simulink model "ConfiguredVirtualVehicleModel"  (R2025b)
settings: Solver=daessc  StartTime=0  StopTime=2474  FixedStep=.001  RelTol=1e-2  EnableMultiTasking=on
StopFcn:
  | %toc
undefined symbols (not defined in the file or in its folder): AccelOvrCmd, CtrlTcuInitGear, DecelOvrCmd, Disabled, DriverPreviewDist, EnblAccelOvr, EnblDecelCmd, EnblSteerCmd, EnvAbsPrs, EnvAirTemp, EnvGrvty, EnvNomFrictionScaling, EnvNominalGrade, EnvWindVelX, EnvWindVelY, EnvWindVelZ, FTP75, MotoFrmInert, MotoFrmLngth, MotoFrmMass, MotoLowrFrntFrkMass, MotoRearArmLngth, MotoRearArmMass, MotoUpprFrntFrkMass, RiderLkAhdPtDstGain, RiderMass, ScnAccTbl, ScnBrkTbl, ScnCRMaxLatAccel, ScnCRRadius, ScnDLCGateLongPos, ScnDLCLatRef, ScnDLCLatRefOffset, ScnDLCLongRefBpt, ScnDLCLongRefStartPos, ScnDLCVehicleWidth, ScnFHCounterDwellTime, ScnFHInitialDwellTime, ScnFHReturnTime, ScnFHRollRateZeroCross, ScnFHSteerAmp, ScnFHSteerSpeed, ScnISHandwheelRate, ScnISMaxHandwheelAng, ScnISMaxLatAccel, ScnISSteerHoldTime, ScnLongPosBpts, ScnLongVelRef, ScnOvalTrackl, ScnOvalTrackpdst, ScnOvalTrackr, ScnSDDwellTime, ScnSDSteerAmp, ScnSDSteerFreq, ScnSSFinalFreq, ScnSSSteerAmp, ScnSSSweepTime, ScnStartTime, ScnStrgAngTbl, ScnStrgTrqTbl ... (+10)
libraries: simulink x16, vehdynlibscenariocommon x9, sm_lib x6, autolibshared x4, nesl_utility x4, vehdynlibviscommon x3, sim3dgroundtruthsensorlib x2, vehdynlibdriver x2, sharedtransform x1, autolibutils x1, sim3dautolib x1, sim3dlib x1
(part 4 of 6)

== system ConfiguredVirtualVehicleModel/Rider Commands/Rider Commands/Roll angle control ==
  MotoFdbk : Inport
  MotoRef : Inport  Port=2
  GearCmd : Inport  Port=3
  Bus Creator1 : BusCreator  Inputs=5
  Bus Selector : BusSelector  OutputSignals=MSteer
  Bus Selector1 : BusSelector  OutputSignals=SteerOvrCmd,AccelOvrCmd,DecelOvrCmd
  Constant : Constant  Value=false
  Constant1 : Constant  Value=30*pi/180
  Demux : Demux  Outputs=1
  Equal Front Rear Bias : Selector  InputPortWidth=1  IndexOptions=Index vector (dialog)  Indices=[1 1]  OutputSizes=1
  Gain : Gain
  Mux : Mux  Inputs=1
  Rider Steering Control : Subsystem  mask{RiderControlTypePanel=Roll angle control, TrajectoryTypePanel=Oval, RidTrajContG=0.11, RidTrajContGphi=-21.5, RidTrajContGphid=9, RidTrajContGl=1.7, RidTrajContTD=0.1, RidTrajContTL=0.1, RidRollContGphi=-21.5, RidRollContGphid=9, Trajr=15, Trajl=80, Trajpointdist=1, TrajDatFile='Traj.mat'}
      mask prompts: RiderControlTypePanel "Rider control type:"; TrajectoryTypePanel "Trajectory type:"; RidTrajContG "Gain to determine the Target roll angle, RidContG [rad/m]:"; RidTrajContGphi "Gain to follow the Target trajectory, RidContGphi [Nm/rad]:"; RidTrajContGphid "Gain to prevent the vehicle from tipping over, RidContGphid [Nms/rad]:"; RidTrajContGl "Gain that determines the distance to the look ahead point, RidContGl [s]:"; RidTrajContTD "Time constant for 1st order delay, RidContTD [s]:"; RidTrajContTL "Dead time of rider operation, RidContTL [s]:"; RidRollContGphi "Gain to follow the Target trajectory, RidContGphi [Nm/rad]:"; RidRollContGphid "Gain to prevent the vehicle from tipping over, RidContGphid [Nms/rad]:"; Trajr "Trajectory parameter,Trajr [m]:"; Trajl "Trajectory parameter,Trajl [m]:"; Trajpointdist "Trajpdist [m]:"; TrajDatFile "Trajectory data file:"
      mask init:
      | maskObj = Simulink.Mask.get(gcb);
      | 
      | Type_tmp = maskObj.getParameter('RiderControlTypePanel');
      | Type     = Type_tmp.Value;
      | 
      | TrajGroup = maskObj.getDialogControl('RiderTrajectoryControlParamPanel');
      | RollGroup = maskObj.getDialogControl('RiderRollControlParamPanel');
      | 
      | TrajectoryTypePanel = maskObj.getDialogControl('TrajectoryTypeCont');
      | TargetTrajectoryParamGroup = maskObj.getDialogControl('TargetTrajectoryParamGroup');
      | 
      | GroupAll = maskObj.getDialogControl('RiderControlParamGroup');
      | 
      | switch Type
      |     case 'Roll angle control'
      |     TrajGroup.Visible = 'off';
      |     RollGroup.Visible = 'on';
      |     GroupAll.Visible = 'on';
      |     TrajectoryTypePanel.Visible = 'off';
      |     TargetTrajectoryParamGroup.Visible = 'off';
      |     InputConnector('TargetRollAngle','on');
      |     case 'Target trajectory driving - Look ahead point'
      |     TrajGroup.Visible = 'on';
      |     RollGroup.Visible = 'off';
      |     GroupAll.Visible = 'on';
      |     TrajectoryTypePanel.Visible = 'on';
      |     TargetTrajectoryParamGroup.Visible = 'on';
      |     InputConnector('TargetRollAngle','off','Ground');
      | end
      | 
      | switch Type
      |     case 'Oval'
      | % ------------------------------------------------------------------------%
      | %  Create Trajectory
      | % ------------------------------------------------------------------------%
      | % --- Oval --- %
      | % top part %
      | x_straight1 = -Trajl/2:Trajpointdist:Trajl/2;
      | y_straight1 = x_straight1*0;
      | 
      | % bottom part %
      | x_straight2 = -Trajl/2:Trajpointdist:Trajl/2;
      | y_straight2 = x_straight1*0+2*Trajr;
      | 
      | % right part %
      | theta_corner1 = -pi/2:Trajpointdist/Trajr:pi/2;
      | x_corner1     = Trajr*cos(theta_corner1)+Trajl/2;
      | y_corner1     = Trajr*sin(theta_corner1)+Trajr;
      | 
      | % left part %
      | theta_corner2 = pi/2:Trajpointdist/Trajr:3/2*pi;
      | x_corner2     = Trajr*cos(theta_corner2)-Trajl/2;
      | y_corner2     = Trajr*sin(theta_corner2)+Trajr;
      | 
      | % total %
      | x_oval = [x_straight1, x_corner1(2:end), fliplr(x_straight2), x_corner2(2:end)];
      | y_oval = [y_straight1, y_corner1(2:end), fliplr(y_straight2), y_corner2(2:end)];
      | 
      | trackData(1,:) = x_oval;
      | trackData(2,:) = y_oval;
      | trackData(3,:) = y_oval*0;
      | 
      |     case 'User defined'
      | 
      | TmpTraj = load(TrajDatFile);
      | 
      | trackData(1,:) = TmpTraj.TrajX;
      | trackData(2,:) = -TmpTraj.TrajY;
      | trackData(3,:) = TmpTraj.TrajY*0;
      | 
      | end
      mask Callback RiderControlTypePanel:
      | maskObj = Simulink.Mask.get(gcb);
      | 
      | Type_tmp = maskObj.getParameter('RiderControlTypePanel');
      | Type     = Type_tmp.Value;
      | 
      | TrajGroup = maskObj.getDialogControl('RiderTrajectoryControlParamPanel');
      | RollGroup = maskObj.getDialogControl('RiderRollControlParamPanel');
      | 
      | TrajectoryTypePanel = maskObj.getDialogControl('TrajectoryTypeCont');
      | TargetTrajectoryParamGroup = maskObj.getDialogControl('TargetTrajectoryParamGroup');
      | 
      | GroupAll = maskObj.getDialogControl('RiderControlParamGroup');
      | 
      | switch Type
      |     case 'Roll angle control'
      |     set_param([gcb,'/Rider Steering'],'RiderControlTypePanel','Roll angle control')
      |     TrajGroup.Visible = 'off';
      |     RollGroup.Visible = 'on';
      |     GroupAll.Visible = 'on';
      |     TrajectoryTypePanel.Visible = 'off';
      |     TargetTrajectoryParamGroup.Visible = 'off';
      |     InputConnector('TargetRollAngle','on');
      |     case 'Target trajectory driving - Look ahead point'
      |     set_param([gcb,'/Rider Steering'],'RiderControlTypePanel','Target trajectory driving - Look ahead point')
      |     TrajGroup.Visible = 'on';
      |     RollGroup.Visible = 'off';
      |     GroupAll.Visible = 'on';
      |     TrajectoryTypePanel.Visible = 'on';
      |     TargetTrajectoryParamGroup.Visible = 'on';
      |     InputConnector('TargetRollAngle','off','Ground');
      | end
      mask TypeOptions TrajectoryTypePanel: Oval | User defined
      mask Callback TrajectoryTypePanel:
      | maskObj = Simulink.Mask.get(gcb);
      | 
      | Type_tmp = maskObj.getParameter('TrajectoryTypePanel');
      | Type = Type_tmp.Value;
      | 
      | TargetTrajectoryParamOvalPanel = maskObj.getDialogControl('TargetTrajectoryParamOvalPanel');
      | 
      | TargetTrajectoryParamUserDefinedPanel = maskObj.getDialogControl('TargetTrajectoryParamUserDefinedPanel');
      | 
      | TargetTrajectoryParamGroup = maskObj.getDialogControl('TargetTrajectoryParamGroup');
      | 
      | switch Type
      |     case 'Oval'
      |         set_param([gcb,'/Rider Steering'],'TrajectoryTypePanel','Oval')
      |         % TargetTrajectoryParamGroup.Visible = 'on';
      |         TargetTrajectoryParamOvalPanel.Visible = 'on';
      |         TargetTrajectoryParamUserDefinedPanel.Visible = 'off';
      |     case 'User defined'
      |     set_param([gcb,'/Rider Steering'],'TrajectoryTypePanel','User defined')
      |         % TargetTrajectoryParamGroup.Visible = 'on';
      |         TargetTrajectoryParamOvalPanel.Visible = 'off';
      |         TargetTrajectoryParamUserDefinedPanel.Visible = 'on';
      | end
      mask DialogControl RiderOptionsGroup Prompt: Options
      mask DialogControl RiderTrajectoryControlParamPanel Prompt: Control parameters
      mask DialogControl RiderRollControlParamPanel Prompt: Control parameters
      mask DialogControl TargetTrajectoryParamOvalPanel Prompt: Trajectory parameters
      mask DialogControl OvalTrajConfBtn Prompt: Confirm
      mask DialogControl OvalTrajConfBtn Callback:
      | maskObj = Simulink.Mask.get(gcb);
      | 
      | Trajr_tmp          = maskObj.getParameter('Trajr');
      | Trajr              = str2num(Trajr_tmp.Value);
      | Trajl_tmp          = maskObj.getParameter('Trajl');
      | Trajl              = str2num(Trajl_tmp.Value);
      | Trajpointdist_tmp  = maskObj.getParameter('Trajpointdist');
      | Trajpointdist      = str2num(Trajpointdist_tmp.Value);
      | 
      | % ------------------------------------------------------------------------%
      | %  Create Trajectory
      | % ------------------------------------------------------------------------%
      | % --- Oval --- %
      | % top part %
      | x_straight1 = -Trajl/2:Trajpointdist:Trajl/2;
      | y_straight1 = x_straight1*0;
      | 
      | % bottom part %
      | x_straight2 = -Trajl/2:Trajpointdist:Trajl/2;
      | y_straight2 = x_straight1*0+2*Trajr;
      | 
      | % right part %
      | theta_corner1 = -pi/2:Trajpointdist/Trajr:pi/2;
      | x_corner1     = Trajr*cos(theta_corner1)+Trajl/2;
      | y_corner1     = Trajr*sin(theta_corner1)+Trajr;
      | 
      | % left part %
      | theta_corner2 = pi/2:Trajpointdist/Trajr:3/2*pi;
      | x_corner2     = Trajr*cos(theta_corner2)-Trajl/2;
      | y_corner2     = Trajr*sin(theta_corner2)+Trajr;
      | 
      | % total %
      | x_oval = [x_straight1, x_corner1(2:end), fliplr(x_straight2), x_corner2(2:end)];
      | y_oval = [y_straight1, y_corner1(2:end), fliplr(y_straight2), y_corner2(2:end)];
      | 
      | figure;
      | plot(x_oval, -y_oval);
      | axis equal;
      | grid on;
      | xlabel('Coordinate X [m]');
      | ylabel('Coordinate Y [m]');
      | title('Oval target trajectory');
      | set(gca,'YDir','reverse')
      mask DialogControl TargetTrajectoryParamUserDefinedPanel Prompt: Trajectory parameters
      mask DialogControl UserDefinedTrajConfBtn Prompt: Confirm
      mask DialogControl UserDefinedTrajConfBtn Callback:
      | maskObj = Simulink.Mask.get(gcb);
      | 
      | File_tmp = maskObj.getParameter('TrajDatFile');
      | File     = replace(File_tmp.Value,'''','');
      | 
      | TmpTraj = load(File);
      | 
      | figure;
      | plot(TmpTraj.TrajX, TmpTraj.TrajY);
      | grid on;
      | axis equal;
      | xlabel('Coordinate X [m]');
      | ylabel('Coordinate Y [m]');
      | title('User defined target trajectory');
      | set(gca,'YDir','reverse');
  Signal Specification{,1..3} (4 alike) : SignalSpecification  Unit=1
  Signal Specification4 : SignalSpecification  Unit=N*m
  Terminator : Terminator
  Rider : Outport  VectorParamsAs1DForOutWhenUnconnected=off
  wires:
  Signal Specification2/1 -> Bus Creator1/4  "GearCmd"
  Bus Selector1/3 -> Signal Specification1/1  "<DecelOvrCmd>"
  Bus Creator1/1 -> Rider/1
  Bus Selector1/2 -> Signal Specification/1  "<AccelOvrCmd>"
  MotoFdbk/1 -> Rider Steering Control/1(sensors)
  Signal Specification/1 -> Bus Creator1/2  "AccelCmd"
  Equal Front Rear Bias/1 -> Bus Creator1/3  "DecelCmd"
  Constant/1 -> Bus Creator1/5  "IgnSwtch"
  MotoRef/1 -> Bus Selector1/1
  GearCmd/1 -> Signal Specification2/1
  Bus Selector1/1 -> Signal Specification3/1  "<SteerOvrCmd>"
  Rider Steering Control/1(RiderInfo) -> Bus Selector/1  "SteerCmd"
  Signal Specification1/1 -> Equal Front Rear Bias/1  "DecelCmd"
  Bus Selector/1 -> Mux/1  "<MSteer>"
  Mux/1 -> Demux/1
  Signal Specification4/1 -> Bus Creator1/1  "SteerCmd"
  Signal Specification3/1 -> Terminator/1  "SteerCmd"
  Constant1/1 -> Rider Steering Control/2(TargetRollAngle)
  Gain/1 -> Signal Specification4/1
  Demux/1 -> Gain/1  "SteerCmd"

== system ConfiguredVirtualVehicleModel/Rider Commands/Rider Commands/Target trajectory following - Look ahead point ==
  MotoFdbk : Inport
  MotoRef : Inport  Port=2
  Env : Inport  Port=3
  Bus Creator1 : BusCreator  Inputs=5
  Bus Selector : BusSelector  OutputSignals=MSteer
  Bus Selector1 : BusSelector  OutputSignals=SteerOvrCmd,LngRef,EnblAccelOvr,AccelOvrCmd,AccelHld,AccelZero,EnblDecelCmd,DecelOvrCmd,DecelHld,DecelZero
  Bus Selector2 : BusSelector  OutputSignals=Body.BdyFrm.Cg.Vel.xdot
  Bus Selector3 : BusSelector  OutputSignals=Grade
  Constant : Constant  Value=false
  Demux : Demux  Outputs=1
  Equal Front Rear Bias : Selector  InputPortWidth=1  IndexOptions=Index vector (dialog)  Indices=[1 1]  OutputSizes=1
  Gain : Gain
  Longitudinal Driver : autolibshared/Longitudinal Driver  extAccelOvr=on  extDecelOvr=on  extAccelHld=on  extDecelHld=on  extAccelZero=on  extDecelZero=on  cntrlType=Predictive  shftType=Reverse, Neutral, Drive  velUnits=m/s  gearOut=on  Kp=5  Ki=5  Kff=.1  Kg=0  VehVelVec=[0 100]  KffVec=[.1 .1]  KpVec=[10 10]  KiVec=[5 5]  KgVec=[0 0]  m=MotoFrmMass+MotoUpprFrntFrkMass+MotoLowrFrntFrkMass+MotoRearArmMass+RiderMass  Kpt=DriverTractiveForce  tau=DriverTimeConst  L=DriverPreviewDist  aR=DriverRollRes  bR=DriverDrivelineRes  cR=DriverAeroRes  g=EnvGrvty  vnom=5  Kaw=1  tauerr=.1  tauPt=2  GearInit=DriverInitialGear  tShift=DriverShiftTime  pdlVec=[0.1 0.4 0.5 0.9]  upShftTbl=[-1 12.9375 26.4375 39.9375 51.18749999999999 62.4375 72.84375 83.25;-1 16.3125 29.8125 43.3125 54.5624 65.8125 76.78125 87.75;-1 19.6875 33.1875 46.68749999999999 57.9375 69.1875 80.71875 92.25;-1 33 52.5 77.25 100.5 138.75 161.875 185]  dwnShftTbl=[1 9.5625 23.0625 36.5625 47.8125 59.0625 68.90625 78.75;1 12.9375 26.4375 39.9375 51.18749999999999 62.4375 72.84375 83.25;1 16.3125 29.8125 43.3125 54.562499 65.8125 76.78125 87.75;1 19.6875 33.1875 46.68749999999999 57.9375 69.1875 80.71875 92.25]  tClutch=.5  tRev=.5  tPark=120  aMode=6  UpGearVec="[0  1  2  3  4  5  6  7]"  DownGearVec="[1  2  3  4  5  6  7  8]"
  Mux : Mux  Inputs=1
  Rider Steering Control : vehdynlibscenariocommon/Rider Steering Control  RiderControlTypePanel=Target trajectory driving - Look ahead point  RidTrajContG=RiderTrgtRollAngGain  RidTrajContGphi=RiderTrgtTrajGain  RidTrajContGphid=RiderPrevTipOvrGain  RidTrajContGl=1.7  RidTrajContTD=RiderFrstOdrTimeCnst  RidTrajContTL=RiderOpDeadTime  RidRollContGphi=-21.5  RidRollContGphid=9
  Signal Specification3 : SignalSpecification  Unit=rad
  Signal Specification4 : SignalSpecification  Unit=N*m
  Terminator : Terminator
  Terminator2 : Terminator
  Unit Conversion1 : UnitConversion
  Rider : Outport  VectorParamsAs1DForOutWhenUnconnected=off
  wires:
  Bus Creator1/1 -> Rider/1
  MotoFdbk/1 -> Bus Selector2/1, Rider Steering Control/1
  Longitudinal Driver/2 -> Bus Creator1/2  "AccelCmd"
  Equal Front Rear Bias/1 -> Bus Creator1/3  "DecelCmd"
  Constant/1 -> Bus Creator1/5  "IgnSwtch"
  Bus Selector1/1 -> Signal Specification3/1  "<SteerOvrCmd>"
  Rider Steering Control/1 -> Bus Selector/1  "SteerCmd"
  Longitudinal Driver/3 -> Equal Front Rear Bias/1  "DecelCmd"
  Bus Selector/1 -> Mux/1  "<MSteer>"
  Mux/1 -> Demux/1
  Signal Specification4/1 -> Bus Creator1/1  "SteerCmd"
  Signal Specification3/1 -> Terminator/1  "SteerCmd"
  Bus Selector1/8 -> Longitudinal Driver/7  "<DecelOvrCmd>"
  Bus Selector1/6 -> Longitudinal Driver/5  "<AccelZero>"
  Bus Selector1/4 -> Longitudinal Driver/3  "<AccelOvrCmd>"
  Bus Selector1/10 -> Longitudinal Driver/9  "<DecelZero>"
  Bus Selector1/5 -> Longitudinal Driver/4  "<AccelHld>"
  MotoRef/1 -> Bus Selector1/1, Rider Steering Control/2
  Bus Selector1/2 -> Unit Conversion1/1  "<LngRef>"
  Bus Selector1/7 -> Longitudinal Driver/6  "<EnblDecelCmd>"
  Bus Selector1/3 -> Longitudinal Driver/2  "<EnblAccelOvr>"
  Bus Selector1/9 -> Longitudinal Driver/8  "<DecelHld>"
  Unit Conversion1/1 -> Longitudinal Driver/1
  Longitudinal Driver/4 -> Bus Creator1/4  "GearCmd"
  Longitudinal Driver/1 -> Terminator2/1
  Bus Selector3/1 -> Longitudinal Driver/11  "<Grade>"
  Env/1 -> Bus Selector3/1
  Bus Selector2/1 -> Longitudinal Driver/10  "<xdot>"
  Gain/1 -> Signal Specification4/1
  Demux/1 -> Gain/1

== system ConfiguredVirtualVehicleModel/Rider Commands/Torque Control/AngleToTorque ==
  MotoFdbk : Inport
  RiderInput : Inport  Port=2
  Bus Creator : BusCreator  Inputs=5
  Bus Selector : BusSelector  OutputSignals=Steer.Genrl.Ang.thetasteer
  Bus Selector1 : BusSelector  OutputSignals=SteerCmd
  Bus Selector2 : BusSelector  OutputSignals=AccelCmd,DecelCmd,GearCmd,IgnSwtch
  Torque Control : vehdynlibsteering/Steering System/Steer by Angle  SystemSampleTime=-1  VariantActivationTime=update diagram  EmptyChoice=off  PassThrough=off  PassThroughVariantControl=(default)  EmptyChoiceVariantControl=(default)  AllowFlexibleInterface=on  Latency=0  AutoFrameSizeCalculation=off
  Rider : Outport
  wires:
  Bus Selector/1 -> Torque Control/2  "<thetasteer>"
  MotoFdbk/1 -> Bus Selector/1
  Bus Selector1/1 -> Torque Control/1  "<SteerCmd>"
  RiderInput/1 -> Bus Selector2/1, Bus Selector1/1
  Bus Selector2/1 -> Bus Creator/2  "<AccelCmd>"
  Bus Selector2/2 -> Bus Creator/3  "<DecelCmd>"
  Bus Selector2/3 -> Bus Creator/4  "<GearCmd>"
  Bus Selector2/4 -> Bus Creator/5  "<IgnSwtch>"
  Torque Control/1 -> Bus Creator/1  "SteerCmd"
  Bus Creator/1 -> Rider/1

== system ConfiguredVirtualVehicleModel/Rider Commands/Torque Control/Look ahead point model ==
  MotoFdbk : Inport
  RiderInput : Inport  Port=2
  MotoRef : Inport  Port=3
  Terminator : Terminator
  Terminator1 : Terminator
  Rider : Outport
  wires:
  MotoFdbk/1 -> Terminator/1
  RiderInput/1 -> Rider/1
  MotoRef/1 -> Terminator1/1

== system ConfiguredVirtualVehicleModel/Rider Commands/Torque Control/NoTorqueControl ==
  MotoFdbk : Inport
  RiderInput : Inport  Port=2
  MotoRef : Inport  Port=3
  Terminator : Terminator
  Terminator1 : Terminator
  Rider : Outport
  wires:
  MotoFdbk/1 -> Terminator/1
  RiderInput/1 -> Rider/1
  MotoRef/1 -> Terminator1/1

== system ConfiguredVirtualVehicleModel/Rider Commands/Torque Control/PID Control ==
  MotoFdbk : Inport
  RiderInput : Inport  Port=2
  MotoRef : Inport  Port=3
  Terminator : Terminator
  Terminator1 : Terminator
  Rider : Outport
  wires:
  MotoFdbk/1 -> Terminator/1
  RiderInput/1 -> Rider/1
  MotoRef/1 -> Terminator1/1

== system ConfiguredVirtualVehicleModel/Visualization/ISO 15037-1:2006/Disabled ==
  VehFdbk : Inport
  Terminator1 : Terminator
  wires:
  VehFdbk/1 -> Terminator1/1

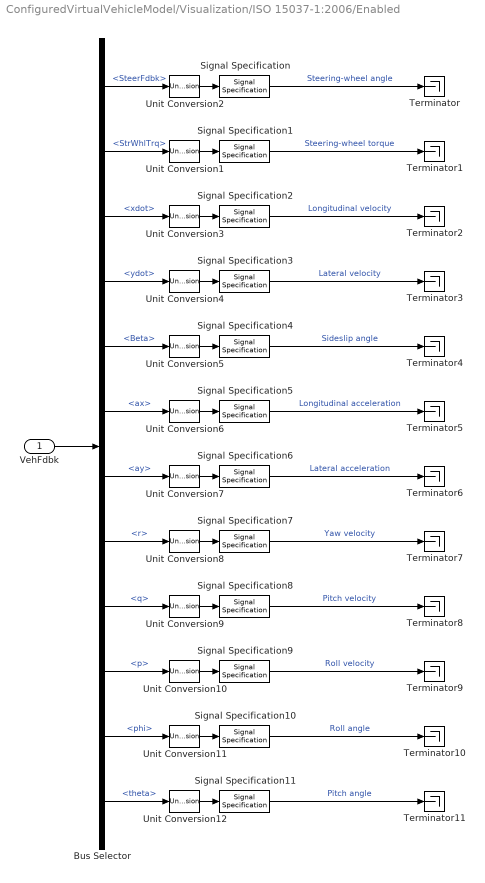
== system ConfiguredVirtualVehicleModel/Visualization/ISO 15037-1:2006/Enabled ==
  VehFdbk : Inport
  Bus Selector : BusSelector  OutputSignals=Rider.SteerFdbk,Steering.StrWhlTrq,Body.BdyFrm.Cg.Vel.xdot,Body.BdyFrm.Cg.Vel.ydot,Body.BdyFrm.Cg.Ang.Beta,Body.BdyFrm.Cg.Acc.ax,Body.BdyFrm.Cg.Acc.ay,Body.BdyFrm.Cg.AngVel.r,Body.BdyFrm.Cg.AngVel.q,Body.BdyFrm.Cg.AngVel.p,Body.InertFrm.Cg.Ang.phi,Body.InertFrm.Cg.Ang.theta
  Signal Specification{,4,10..11} (4 alike) : SignalSpecification  Unit=deg
  Signal Specification1 : SignalSpecification  Unit=N*m
  Signal Specification2 : SignalSpecification  Unit=km/h
  Signal Specification3 : SignalSpecification  Unit=m/s
  Signal Specification5 : SignalSpecification  Unit=m/s^2
  Signal Specification6 : SignalSpecification  Unit=m/s^2
  Signal Specification7 : SignalSpecification  Unit=deg/s
  Signal Specification8 : SignalSpecification  Unit=deg/s
  Signal Specification9 : SignalSpecification  Unit=deg/s
  Terminator{,1..11} (12 alike) : Terminator
  Unit Conversion{1..12} (12 alike) : UnitConversion
  wires:
  Bus Selector/12 -> Unit Conversion12/1  "<theta>"
  Signal Specification11/1 -> Terminator11/1  "Pitch angle"
  Unit Conversion12/1 -> Signal Specification11/1
  Bus Selector/11 -> Unit Conversion11/1  "<phi>"
  Unit Conversion11/1 -> Signal Specification10/1
  Signal Specification10/1 -> Terminator10/1  "Roll angle"
  Bus Selector/10 -> Unit Conversion10/1  "<p>"
  Signal Specification9/1 -> Terminator9/1  "Roll velocity"
  Unit Conversion10/1 -> Signal Specification9/1
  Bus Selector/9 -> Unit Conversion9/1  "<q>"
  Unit Conversion9/1 -> Signal Specification8/1
  Signal Specification8/1 -> Terminator8/1  "Pitch velocity"
  Bus Selector/8 -> Unit Conversion8/1  "<r>"
  Signal Specification7/1 -> Terminator7/1  "Yaw velocity"
  Unit Conversion8/1 -> Signal Specification7/1
  Bus Selector/7 -> Unit Conversion7/1  "<ay>"
  Unit Conversion7/1 -> Signal Specification6/1
  Signal Specification6/1 -> Terminator6/1  "Lateral acceleration"
  Bus Selector/6 -> Unit Conversion6/1  "<ax>"
  Signal Specification5/1 -> Terminator5/1  "Longitudinal acceleration"
  Unit Conversion6/1 -> Signal Specification5/1
  Bus Selector/5 -> Unit Conversion5/1  "<Beta>"
  Unit Conversion5/1 -> Signal Specification4/1
  Signal Specification4/1 -> Terminator4/1  "Sideslip angle"
  Bus Selector/4 -> Unit Conversion4/1  "<ydot>"
  Signal Specification3/1 -> Terminator3/1  "Lateral velocity"
  Unit Conversion4/1 -> Signal Specification3/1
  Bus Selector/3 -> Unit Conversion3/1  "<xdot>"
  Unit Conversion3/1 -> Signal Specification2/1
  Signal Specification2/1 -> Terminator2/1  "Longitudinal velocity"
  Signal Specification1/1 -> Terminator1/1  "Steering-wheel torque"
  Unit Conversion1/1 -> Signal Specification1/1
  Bus Selector/2 -> Unit Conversion1/1  "<StrWhlTrq>"
  Signal Specification/1 -> Terminator/1  "Steering-wheel angle"
  Unit Conversion2/1 -> Signal Specification/1
  VehFdbk/1 -> Bus Selector/1
  Bus Selector/1 -> Unit Conversion2/1  "<SteerFdbk>"

== system ConfiguredVirtualVehicleModel/Visualization/Performance Signal Routing/Performance Calculations ==
  VehSpd : Inport
  FuelVolFlow : Inport  Port=2
  BattPwr : Inport  Port=3
  Add : Sum
  Divide : Product  Inputs=*/
  Divide1 : Product  Inputs=*/
  Divide2 : Product  Inputs=*/
  Integrator : Integrator
  Integrator1 : Integrator
  L/100 Km Calc : Product  Inputs=/*
  Product : Product
  Rate Transition3 : RateTransition  Deterministic=off
  Saturation : Saturate  UpperLimit=Inf  LowerLimit=0.001  ZeroCross=off
  Saturation1 : Saturate  UpperLimit=Inf  LowerLimit=1e-3  ZeroCross=off
  Signal Specification5 : SignalSpecification  Unit=m/s
  Sqrt : Sqrt
  US EPA kwh/USgal equivalent : Constant  Value=33.7
  US MPG Calc : Product  Inputs=*/
  Unit Conversion5 : UnitConversion
  m to 100Km : Gain  Gain=1/1000/100
  m to mile : Gain  Gain=0.000621371
  m^3 per gal : Gain  Gain=0.00378541
  m^3 to L : Gain  Gain=1000
  m^3 to US Gal : Gain  Gain=264.172
  s per h : Constant  Value=3600
  w per kw : Constant  Value=1000
  US MPG : Outport  VectorParamsAs1DForOutWhenUnconnected=off
  L/100Km : Outport  Port=2  VectorParamsAs1DForOutWhenUnconnected=off
  wires:
  m^3 to US Gal/1 -> Saturation1/1
  m^3 to L/1 -> L/100 Km Calc/2
  Integrator/1 -> m to mile/1, m to 100Km/1
  m to mile/1 -> US MPG Calc/1
  FuelVolFlow/1 -> Add/1
  Integrator1/1 -> m^3 to US Gal/1, m^3 to L/1
  Saturation/1 -> L/100 Km Calc/1
  m to 100Km/1 -> Saturation/1
  L/100 Km Calc/1 -> L/100Km/1  "L/100Km"
  US MPG Calc/1 -> Rate Transition3/1
  Saturation1/1 -> US MPG Calc/2
  Rate Transition3/1 -> US MPG/1  "US MPG"
  w per kw/1 -> Divide/2
  Divide/1 -> Divide2/1
  Divide2/1 -> Divide1/1
  s per h/1 -> Divide1/2
  Divide1/1 -> m^3 per gal/1
  Add/1 -> Integrator1/1
  m^3 per gal/1 -> Add/2
  US EPA kwh/USgal equivalent/1 -> Divide2/2
  BattPwr/1 -> Divide/1
  Sqrt/1 -> Integrator/1
  Product/1 -> Sqrt/1
  Signal Specification5/1 -> Product/2, Product/1
  Unit Conversion5/1 -> Signal Specification5/1
  VehSpd/1 -> Unit Conversion5/1

== system ConfiguredVirtualVehicleModel/Visualization/Scope Type/DLC ==
  VehFdbk : Inport
  Vis : Inport  Port=2
  Bus Creator : BusCreator  Inputs=3
  Bus Selector3 : BusSelector  OutputSignals=Body.InertFrm.Cg.Disp.X,Body.InertFrm.Cg.Disp.Z
  Bus Selector4 : BusSelector  OutputSignals=LeftBnd,RightBnd,LtrlRef
  Lane Change : Scope
      settings: Title=Double Lane Change: Lateral Displacement  ActiveDisplayYMinimum=-3.28469  ActiveDisplayYMaximum=6.06905  YLabel=Lateral Displacement [m] (positive = right direction)  DataLoggingSaveFormat=Array
  Mux1 : Mux  Inputs=3
  Rate Transition : RateTransition  OutPortSampleTime=.1
  Rate Transition3 : RateTransition  OutPortSampleTime=.1
  Signal Copy : SignalConversion  OverrideOpt=off
  Signal Copy1 : SignalConversion  OverrideOpt=off
  Signal Copy2 : SignalConversion  OverrideOpt=off
  Ref : Outport  VectorParamsAs1DForOutWhenUnconnected=off
  wires:
  VehFdbk/1 -> Bus Selector3/1
  Vis/1 -> Bus Selector4/1
  Bus Creator/1 -> Ref/1
  Bus Selector3/2 -> Signal Copy2/1  "<Z>"
  Signal Copy/1 -> Bus Creator/2  "YRef"
  Signal Copy1/1 -> Bus Creator/1  "XRef"
  Signal Copy2/1 -> Bus Creator/3  "ZRef"
  Rate Transition3/1 -> Mux1/2  "Right Boundary"
  Bus Selector4/3 -> Signal Copy/1, Mux1/3  "<LtrlRef>"
  Mux1/1 -> Lane Change/1
  Bus Selector4/1 -> Rate Transition/1  "<LeftBnd>"
  Rate Transition/1 -> Mux1/1  "Left Boundary"
  Bus Selector4/2 -> Rate Transition3/1  "<RightBnd>"
  Bus Selector3/1 -> Signal Copy1/1  "<X>"

== system ConfiguredVirtualVehicleModel/Visualization/Scope Type/None ==
  VehFdbk : Inport
  Vis : Inport  Port=2
  Bus Selector2 : BusSelector  OutputSignals=Steer.Genrl.Ang.thetasteer
  Bus Selector9 : BusSelector  OutputSignals=Body.BdyFrm.Cg.AngVel.r
  Signal Specification3 : SignalSpecification  Unit=deg/s
  Unit Conversion4 : UnitConversion
  Yaw Rate and Steer : Scope  NumInputPorts=2
      settings: ActiveDisplayYMinimum=-112.49987  ActiveDisplayYMaximum=112.49996
  Ref : Outport  VectorParamsAs1DForOutWhenUnconnected=off
  wires:
  Bus Selector9/1 -> Unit Conversion4/1  "<r>"
  Signal Specification3/1 -> Yaw Rate and Steer/1
  Unit Conversion4/1 -> Signal Specification3/1
  VehFdbk/1 -> Bus Selector2/1, Bus Selector9/1  "VehFdbk"
  Bus Selector2/1 -> Yaw Rate and Steer/2  "<thetasteer>"
  Vis/1 -> Ref/1

== system ConfiguredVirtualVehicleModel/Visualization/Scope Type/XYZ ==
  VehFdbk : Inport
  Vis : Inport  Port=2
  Terminator : Terminator
  Ref : Outport  VectorParamsAs1DForOutWhenUnconnected=off
  wires:
  Vis/1 -> Ref/1
  VehFdbk/1 -> Terminator/1

== system ConfiguredVirtualVehicleModel/Visualization/Vehicle XY Plotter/Disabled ==

== system ConfiguredVirtualVehicleModel/Visualization/Vehicle XY Plotter/XY View ==
  Bus Element In2 : Inport  PortName=VehFdbk
  Bus Selector1 : BusSelector  OutputSignals=Body.InertFrm.Cg.Ang.phi,Body.InertFrm.Cg.Ang.theta,Body.InertFrm.Cg.Ang.psi  OutputAsBus=on
  Bus Selector2 : BusSelector  OutputSignals=Wheels.FrontTire.Fx,Wheels.RearTire.Fx
  Bus Selector3 : BusSelector  OutputSignals=Wheels.FrontTire.Fy,Wheels.RearTire.Fy
  Bus Selector5 : BusSelector  OutputSignals=Wheels.FrontTire.Alpha,Wheels.RearTire.Alpha
  Bus Selector6 : BusSelector  OutputSignals=Body.InertFrm.Cg.Disp.X,Body.InertFrm.Cg.Disp.Y,Body.InertFrm.Cg.Disp.Z  OutputAsBus=on
  Bus Selector7 : BusSelector  OutputSignals=Body.InertFrm.Cg.Vel.Xdot,Body.InertFrm.Cg.Vel.Ydot,Body.InertFrm.Cg.Vel.Zdot  OutputAsBus=on
  Bus Selector9 : BusSelector  OutputSignals=Driveline.EngSpd,Driveline.EMSpd,Driveline.Gear
  Bus to Vector : BusToVector
  Bus to Vector1 : BusToVector
  Bus to Vector2 : BusToVector
  Max : MinMax  Function=max  Inputs=2
  Multi-Track XY Plotter : vehdynlibviscommon/Multi-Track XY Plotter  numTrack=Single track  extRef=off  extStats=on  extTireF=on  a=1.5  b=1.5  w=0  figBorder=10  bufferSize=1024  velNorm=5  tireFNorm=1000  pltDT=.1
      settings: LibrarySourceBlock=vehdynlibviscommon/Vehicle XY Plot Configuration
  Mux{,1..3} (4 alike) : Mux  Inputs=2
  Unary Minus : UnaryMinus
  wires:
  Bus Selector7/1 -> Bus to Vector1/1
  Bus to Vector1/1 -> Multi-Track XY Plotter/3
  Bus Selector2/1 -> Mux1/1  "<Fx>"
  Bus Selector1/1 -> Bus to Vector2/1
  Bus Selector9/1 -> Max/1  "<EngSpd>"
  Bus to Vector/1 -> Multi-Track XY Plotter/1
  Bus Selector6/1 -> Bus to Vector/1
  Bus to Vector2/1 -> Multi-Track XY Plotter/2
  Bus Element In2/1 -> Bus Selector3/1, Bus Selector2/1, Bus Selector9/1, Bus Selector5/1, Bus Selector7/1, Bus Selector1/1, Bus Selector6/1  "VehFdbk"
  Mux3/1 -> Multi-Track XY Plotter/4
  Mux1/1 -> Multi-Track XY Plotter/6
  Mux2/1 -> Unary Minus/1
  Max/1 -> Mux/1
  Bus Selector9/2 -> Max/2  "<EMSpd>"
  Mux/1 -> Multi-Track XY Plotter/5
  Bus Selector9/3 -> Mux/2  "<Gear>"
  Bus Selector2/2 -> Mux1/2  "<Fx>"
  Bus Selector3/2 -> Mux2/2  "<Fy>"
  Bus Selector3/1 -> Mux2/1  "<Fy>"
  Bus Selector5/1 -> Mux3/1  "<Alpha>"
  Bus Selector5/2 -> Mux3/2  "<Alpha>"
  Unary Minus/1 -> Multi-Track XY Plotter/7

== system ConfiguredVirtualVehicleModel/Visualization/Vehicle XY Plotter/XY View Ref ==
  Bus Element In2 : Inport  PortName=VehFdbk
  Bus Element In1 : Inport  Port=2  PortName=Ref  Element=YRef
  Bus Element In3 : Inport  Port=2  PortName=Ref  Element=XRef
  Bus Selector1 : BusSelector  OutputSignals=Body.InertFrm.Cg.Ang.phi,Body.InertFrm.Cg.Ang.theta,Body.InertFrm.Cg.Ang.psi  OutputAsBus=on
  Bus Selector10 : BusSelector  OutputSignals=Wheels.FrontTire.Fx,Wheels.RearTire.Fx,Wheels.FrontTire.Fy,Wheels.RearTire.Fy
  Bus Selector5 : BusSelector  OutputSignals=Steer.Genrl.Ang.thetasteer,Wheels.RearTire.Alpha
  Bus Selector6 : BusSelector  OutputSignals=Body.InertFrm.Cg.Disp.X,Body.InertFrm.Cg.Disp.Y,Body.InertFrm.Cg.Disp.Z  OutputAsBus=on
  Bus Selector7 : BusSelector  OutputSignals=Body.InertFrm.Cg.Vel.Xdot,Body.InertFrm.Cg.Vel.Ydot,Body.InertFrm.Cg.Vel.Zdot  OutputAsBus=on
  Bus Selector9 : BusSelector  OutputSignals=Driveline.EngSpd,Driveline.EMSpd,Driveline.Gear
  Bus to Vector : BusToVector
  Bus to Vector1 : BusToVector
  Bus to Vector2 : BusToVector
  Ground1 : Ground
  Max : MinMax  Function=max  Inputs=2
  Multi-Track XY Plotter : vehdynlibviscommon/Multi-Track XY Plotter  numTrack=Single track  extRef=on  extStats=on  extTireF=on  a=1.5  b=1.5  w=0  figBorder=10  bufferSize=1024  velNorm=5  tireFNorm=1000  pltDT=.1
      settings: LibrarySourceBlock=vehdynlibviscommon/Vehicle XY Plot Configuration
  Mux : Mux  Inputs=3
  Mux{1..4} (4 alike) : Mux  Inputs=2
  Unary Minus : UnaryMinus
  wires:
  Bus Selector7/1 -> Bus to Vector1/1
  Ground1/1 -> Mux/3
  Mux2/1 -> Unary Minus/1
  Bus to Vector1/1 -> Multi-Track XY Plotter/3
  Mux1/1 -> Multi-Track XY Plotter/7
  Bus Selector1/1 -> Bus to Vector2/1
  Bus Element In1/1 -> Mux/2
  Mux4/1 -> Multi-Track XY Plotter/6
  Bus Element In3/1 -> Mux/1
  Mux/1 -> Multi-Track XY Plotter/5
  Bus to Vector/1 -> Multi-Track XY Plotter/1
  Bus Selector6/1 -> Bus to Vector/1
  Bus to Vector2/1 -> Multi-Track XY Plotter/2
  Bus Selector5/1 -> Mux3/1  "<thetasteer>"
  Mux3/1 -> Multi-Track XY Plotter/4
  Bus Selector5/2 -> Mux3/2  "<Alpha>"
  Bus Selector10/1 -> Mux1/1  "<Fx>"
  Bus Selector10/2 -> Mux1/2  "<Fx>"
  Bus Selector10/3 -> Mux2/1  "<Fy>"
  Bus Selector10/4 -> Mux2/2  "<Fy>"
  Unary Minus/1 -> Multi-Track XY Plotter/8
  Bus Selector9/3 -> Mux4/2  "<Gear>"
  Bus Selector9/1 -> Max/1  "<EngSpd>"
  Bus Selector9/2 -> Max/2  "<EMSpd>"
  Max/1 -> Mux4/1
  Bus Element In2/1 -> Bus Selector9/1, Bus Selector10/1, Bus Selector5/1, Bus Selector7/1, Bus Selector1/1, Bus Selector6/1  "VehFdbk"

== system ConfiguredVirtualVehicleModel/Environment/Friction/Varying Friction/Road Track Friction ==
  XWhl : Inport
  YWhl : Inport  Port=2
  Cg : Inport  Port=3
  2D Lookup Tbl for Scaling Fctr (Lambda) : Subsystem  TreatAsAtomicUnit=on
      mask init:
      | [~]=vehdynicon('vehdynblk',gcb);
  Bus Selector : BusSelector  OutputSignals=X,Y
  Cnst Lambda : Constant  Value=ones(2,1).*lambda_g
  Constant1 : Constant  Value=SplitLambdaTrck
  Creating Inertial Frm Bpt : Subsystem
  En at t = 0 : Subsystem
  "Lambda (t = 0) " : Memory  InitialCondition=ones(2,1).*lambda_g  InheritSampleTime=on
  Switch : Switch  Criteria=u2 > Threshold  ZeroCross=off  SaturateOnIntegerOverflow=off  InputSameDT=off
  FricCoeffLambda : Outport
  wires:
  YWhl/1 -> 2D Lookup Tbl for Scaling Fctr (Lambda)/2(YWhl)
  XWhl/1 -> 2D Lookup Tbl for Scaling Fctr (Lambda)/1(XWhl)
  2D Lookup Tbl for Scaling Fctr (Lambda)/1(Lambda for each whl) -> Switch/1
  "Lambda (t = 0) "/1 -> FricCoeffLambda/1
  Switch/1 -> "Lambda (t = 0) "/1
  Cnst Lambda/1 -> Switch/3
  Constant1/1 -> Switch/2
  Cg/1 -> Bus Selector/1
  Creating Inertial Frm Bpt/1(XBpt) -> 2D Lookup Tbl for Scaling Fctr (Lambda)/3(XBpt)
  Creating Inertial Frm Bpt/2(YBpt) -> 2D Lookup Tbl for Scaling Fctr (Lambda)/4(YBpt)
  Bus Selector/1 -> Creating Inertial Frm Bpt/1(XCg)  "<X>"
  Bus Selector/2 -> Creating Inertial Frm Bpt/2(YCg)  "<Y>"
  En at t = 0/1(Out1) -> Creating Inertial Frm Bpt/Enable

== system ConfiguredVirtualVehicleModel/Environment/Friction/Varying Friction/Wheel Coordinates ==
  FrntAxlX : Inport
  RearAxlX : Inport  Port=2
  FrntAxlY : Inport  Port=3
  RearAxlY : Inport  Port=4
  Matrix Concatenate : Concatenate  Mode=Multidimensional array
  Matrix Concatenate1 : Concatenate  Mode=Multidimensional array
  XWhl : Outport
  YWhl : Outport  Port=2
  wires:
  Matrix Concatenate/1 -> XWhl/1
  FrntAxlX/1 -> Matrix Concatenate/1
  Matrix Concatenate1/1 -> YWhl/1
  FrntAxlY/1 -> Matrix Concatenate1/1
  RearAxlY/1 -> Matrix Concatenate1/2
  RearAxlX/1 -> Matrix Concatenate/2

== system ConfiguredVirtualVehicleModel/Environment/Ground Feedback/3D Engine/3D Engine Source ==
  WheelFdbk : Inport
  Multiple Points : Subsystem  VariantControl=terrType==2
  Single Point : Subsystem  VariantControl=terrType ==1
  z : Outport
  DCM : Outport  Port=2

== system ConfiguredVirtualVehicleModel/Motorcycle Vehicle/Hand Levers and Pedals/Hand Levers and Pedals/Brake Pedal ==
  DecelCmd : Inport
  Dead Zone1 : DeadZone  LowerValue=0  UpperValue=.01  ZeroCross=off
  DecelFdbk : Outport
  wires:
  Dead Zone1/1 -> DecelFdbk/1
  DecelCmd/1 -> Dead Zone1/1

== system ConfiguredVirtualVehicleModel/Motorcycle Vehicle/Transmission, Driveline and Brakes/Transmission and Driveline/Driveline ==
  FCpR : Inport
  ThetaFrm : Inport  Port=2
  ThetaArmR : Inport  Port=3
  MBrkR : Inport  Port=4
  AngAWhlR : Inport  Port=5
  DrvSprktTrq : Inport  Port=6
  Chain_Drive : Subsystem  VariantControl=Chain_Drive  ReferencedSubsystem=Chain_Drive
  Info : Outport
  DrvSprktSpd : Outport  Port=2

== system ConfiguredVirtualVehicleModel/Motorcycle Vehicle/Transmission, Driveline and Brakes/Transmission and Driveline/Transmission ==
  EngTrq : Inport
  GearCmd : Inport  Port=2
  EMTrq : Inport  Port=3
  DrvSprktSpd : Inport  Port=4
  ConventionalMotorcycle : Subsystem  VariantControl=ConventionalMotorcycle  ReferencedSubsystem=ConventionalMotorcycle
  EngSpd : Outport
  Gear : Outport  Port=2
  EMSpd : Outport  Port=3
  DrvSprktTrq : Outport  Port=4

== system ConfiguredVirtualVehicleModel/Reference Generator for Motorcycle/3D Engine/3D Engine/Wheel Rotations ==
  MotoFdbk : Inport
  Bus Selector2 : BusSelector  OutputSignals=Wheels.FrontTire.Omega,Wheels.RearTire.Omega
  Constant{4,6..8} (4 alike) : Constant  Value=0  VectorParams1D=off
  Demux : Demux  Outputs=2
  Integrator : Integrator  WrapState=on  WrappedStateUpperValue=2*pi  WrappedStateLowerValue=0  ZeroCross=off
  Mux1 : Mux  Inputs=2
  Rotation : Concatenate  NumInputs=3  Mode=Multidimensional array  ConcatenateDimension=2
  Rotation1 : Concatenate  NumInputs=3  Mode=Multidimensional array  ConcatenateDimension=2
  Front : Outport
  Rear : Outport  Port=2
  wires:
  Constant4/1 -> Rotation1/1
  Mux1/1 -> Integrator/1
  Integrator/1 -> Demux/1
  Demux/1 -> Rotation/2
  Demux/2 -> Rotation1/2
  Constant7/1 -> Rotation/1
  Constant8/1 -> Rotation/3
  Constant6/1 -> Rotation1/3
  Bus Selector2/1 -> Mux1/1  "<Omega>"
  Rotation1/1 -> Rear/1
  Bus Selector2/2 -> Mux1/2  "<Omega>"
  Rotation/1 -> Front/1
  MotoFdbk/1 -> Bus Selector2/1

== system ConfiguredVirtualVehicleModel/Reference Generator for Motorcycle/Reference Router/Steering Command Override/Control Signals ==
  note: 1) Add Subsystem or Model blocks as valid variant choices.
      | 2) You cannot connect blocks at this level. At simulation, connectivity is automatically
      | determined, based on the active variant and port name matching.
  Time : Inport
  Position : Inport  Port=2
  Position-Based Angle : Subsystem  VariantControl=OverrideType==2 && ActType== 2
  Position-Based Torque : Subsystem  VariantControl=OverrideType==1 && ActType== 2
  Time-Based Angle : Subsystem  VariantControl=OverrideType==2 && ActType==1
  Time-Based Torque : Subsystem  VariantControl=OverrideType==1 && ActType== 1
  Steer : Outport

== system ConfiguredVirtualVehicleModel/Reference Generator for Motorcycle/Reference Router/Steering and Accel and Brk Command Override/Control Signals ==
  note: 1) Add Subsystem or Model blocks as valid variant choices.
      | 2) You cannot connect blocks at this level. At simulation, connectivity is automatically
      | determined, based on the active variant and port name matching.
  Time : Inport
  Position : Inport  Port=2
  Position-Based Angle : Subsystem  VariantControl=OverrideType==2 && ActType== 2
  Position-Based Torque : Subsystem  VariantControl=OverrideType==1 && ActType== 2
  Time-Based Angle : Subsystem  VariantControl=OverrideType==2 && ActType==1
  Time-Based Torque : Subsystem  VariantControl=OverrideType==1 && ActType== 1
  Steer : Outport
  Accel : Outport  Port=2
  Brake : Outport  Port=3

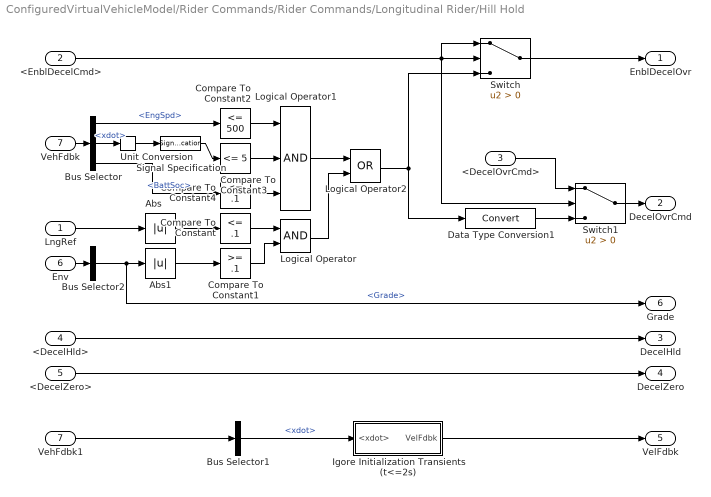
== system ConfiguredVirtualVehicleModel/Rider Commands/Rider Commands/Longitudinal Rider/Hill Hold ==
  LngRef : Inport
  <EnblDecelCmd> : Inport  Port=2
  <DecelOvrCmd> : Inport  Port=3
  <DecelHld> : Inport  Port=4
  <DecelZero> : Inport  Port=5
  Env : Inport  Port=6
  VehFdbk : Inport  Port=7
  Abs : Abs  ZeroCross=off  SaturateOnIntegerOverflow=off
  Abs1 : Abs  ZeroCross=off  SaturateOnIntegerOverflow=off
  Bus Selector : BusSelector  OutputSignals=Engine.EngineInfo.EngSpd,Body.BdyFrm.Cg.Vel.xdot,Battery.BattSoc
  Bus Selector1 : BusSelector  OutputSignals=Body.BdyFrm.Cg.Vel.xdot
  Bus Selector2 : BusSelector  OutputSignals=Grade
  Compare To Constant : simulink/Logic and Bit Operations/Compare To Constant  relop=<=  const=.1  OutDataTypeStr=boolean  ZeroCross=off
  Compare To Constant1 : simulink/Logic and Bit Operations/Compare To Constant  relop=>=  const=.1  OutDataTypeStr=boolean  ZeroCross=off
  Compare To Constant2 : simulink/Logic and Bit Operations/Compare To Constant  relop=<=  const=500  OutDataTypeStr=boolean  ZeroCross=off
  Compare To Constant3 : simulink/Logic and Bit Operations/Compare To Constant  relop=<=  const=5  OutDataTypeStr=boolean  ZeroCross=off
  Compare To Constant4 : simulink/Logic and Bit Operations/Compare To Constant  relop=<=  const=.1  OutDataTypeStr=boolean  ZeroCross=off
  Data Type Conversion1 : DataTypeConversion  SaturateOnIntegerOverflow=off  RndMeth=Floor
  Igore Initialization Transients (t<=2s) : Subsystem
  Logical Operator : Logic  AllPortsSameDT=off  OutDataTypeStr=boolean
  Logical Operator1 : Logic  Inputs=3  AllPortsSameDT=off  OutDataTypeStr=boolean
  Logical Operator2 : Logic  Operator=OR  AllPortsSameDT=off  OutDataTypeStr=boolean
  Signal Specification : SignalSpecification  Unit=m/s
  Switch : Switch  Criteria=u2 > Threshold  SaturateOnIntegerOverflow=off  InputSameDT=off
  Switch1 : Switch  Criteria=u2 > Threshold  SaturateOnIntegerOverflow=off  InputSameDT=off
  Unit Conversion : UnitConversion
  VehFdbk1 : InportShadow  Port=7
  EnblDecelOvr : Outport
  DecelOvrCmd : Outport  Port=2
  DecelHld : Outport  Port=3
  DecelZero : Outport  Port=4
  VelFdbk : Outport  Port=5
  Grade : Outport  Port=6
  wires:
  Logical Operator2/1 -> Switch/3, Data Type Conversion1/1
  LngRef/1 -> Abs/1
  Abs/1 -> Compare To Constant/1
  Compare To Constant/1 -> Logical Operator/1
  Abs1/1 -> Compare To Constant1/1
  Compare To Constant1/1 -> Logical Operator/2
  Compare To Constant2/1 -> Logical Operator1/1
  Compare To Constant3/1 -> Logical Operator1/2
  Logical Operator1/1 -> Logical Operator2/1
  Logical Operator/1 -> Logical Operator2/2
  Compare To Constant4/1 -> Logical Operator1/3
  VehFdbk/1 -> Bus Selector/1
  Bus Selector/1 -> Compare To Constant2/1  "<EngSpd>"
  Bus Selector/2 -> Unit Conversion/1  "<xdot>"
  Bus Selector/3 -> Compare To Constant4/1  "<BattSoc>"
  Data Type Conversion1/1 -> Switch1/3
  <EnblDecelCmd>/1 -> Switch1/2, Switch/1, Switch/2
  Switch/1 -> EnblDecelOvr/1
  <DecelOvrCmd>/1 -> Switch1/1
  Switch1/1 -> DecelOvrCmd/1
  Env/1 -> Bus Selector2/1
  Bus Selector2/1 -> Grade/1, Abs1/1  "<Grade>"
  VehFdbk1/1 -> Bus Selector1/1
  Bus Selector1/1 -> Igore Initialization Transients (t<=2s)/1(<xdot>)  "<xdot>"
  Igore Initialization Transients (t<=2s)/1(VelFdbk) -> VelFdbk/1
  <DecelZero>/1 -> DecelZero/1
  <DecelHld>/1 -> DecelHld/1
  Unit Conversion/1 -> Signal Specification/1
  Signal Specification/1 -> Compare To Constant3/1

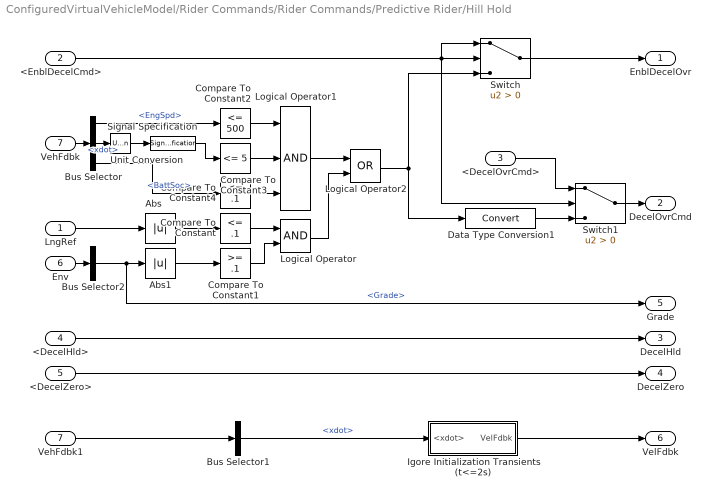
== system ConfiguredVirtualVehicleModel/Rider Commands/Rider Commands/Predictive Rider/Hill Hold ==
  LngRef : Inport
  <EnblDecelCmd> : Inport  Port=2
  <DecelOvrCmd> : Inport  Port=3
  <DecelHld> : Inport  Port=4
  <DecelZero> : Inport  Port=5
  Env : Inport  Port=6
  VehFdbk : Inport  Port=7
  Abs : Abs  ZeroCross=off  SaturateOnIntegerOverflow=off
  Abs1 : Abs  ZeroCross=off  SaturateOnIntegerOverflow=off
  Bus Selector : BusSelector  OutputSignals=Engine.EngineInfo.EngSpd,Body.BdyFrm.Cg.Vel.xdot,Battery.BattSoc
  Bus Selector1 : BusSelector  OutputSignals=Body.BdyFrm.Cg.Vel.xdot
  Bus Selector2 : BusSelector  OutputSignals=Grade
  Compare To Constant : simulink/Logic and Bit Operations/Compare To Constant  relop=<=  const=.1  OutDataTypeStr=boolean  ZeroCross=off
  Compare To Constant1 : simulink/Logic and Bit Operations/Compare To Constant  relop=>=  const=.1  OutDataTypeStr=boolean  ZeroCross=off
  Compare To Constant2 : simulink/Logic and Bit Operations/Compare To Constant  relop=<=  const=500  OutDataTypeStr=boolean  ZeroCross=off
  Compare To Constant3 : simulink/Logic and Bit Operations/Compare To Constant  relop=<=  const=5  OutDataTypeStr=boolean  ZeroCross=off
  Compare To Constant4 : simulink/Logic and Bit Operations/Compare To Constant  relop=<=  const=.1  OutDataTypeStr=boolean  ZeroCross=off
  Data Type Conversion1 : DataTypeConversion  SaturateOnIntegerOverflow=off  RndMeth=Floor
  Igore Initialization Transients (t<=2s) : Subsystem
  Logical Operator : Logic  AllPortsSameDT=off  OutDataTypeStr=boolean
  Logical Operator1 : Logic  Inputs=3  AllPortsSameDT=off  OutDataTypeStr=boolean
  Logical Operator2 : Logic  Operator=OR  AllPortsSameDT=off  OutDataTypeStr=boolean
  Signal Specification : SignalSpecification  Unit=m/s
  Switch : Switch  Criteria=u2 > Threshold  SaturateOnIntegerOverflow=off  InputSameDT=off
  Switch1 : Switch  Criteria=u2 > Threshold  SaturateOnIntegerOverflow=off  InputSameDT=off
  Unit Conversion : UnitConversion
  VehFdbk1 : InportShadow  Port=7
  EnblDecelOvr : Outport
  DecelOvrCmd : Outport  Port=2
  DecelHld : Outport  Port=3
  DecelZero : Outport  Port=4
  Grade : Outport  Port=5
  VelFdbk : Outport  Port=6
  wires:
  Logical Operator2/1 -> Switch/3, Data Type Conversion1/1
  LngRef/1 -> Abs/1
  Abs/1 -> Compare To Constant/1
  Compare To Constant/1 -> Logical Operator/1
  Abs1/1 -> Compare To Constant1/1
  Compare To Constant1/1 -> Logical Operator/2
  Compare To Constant2/1 -> Logical Operator1/1
  Compare To Constant3/1 -> Logical Operator1/2
  Logical Operator1/1 -> Logical Operator2/1
  Logical Operator/1 -> Logical Operator2/2
  Compare To Constant4/1 -> Logical Operator1/3
  VehFdbk/1 -> Bus Selector/1
  Bus Selector/1 -> Compare To Constant2/1  "<EngSpd>"
  Bus Selector/3 -> Compare To Constant4/1  "<BattSoc>"
  Data Type Conversion1/1 -> Switch1/3
  <EnblDecelCmd>/1 -> Switch1/2, Switch/1, Switch/2
  Switch/1 -> EnblDecelOvr/1
  <DecelOvrCmd>/1 -> Switch1/1
  Switch1/1 -> DecelOvrCmd/1
  Env/1 -> Bus Selector2/1
  Bus Selector2/1 -> Grade/1, Abs1/1  "<Grade>"
  VehFdbk1/1 -> Bus Selector1/1
  Bus Selector1/1 -> Igore Initialization Transients (t<=2s)/1(<xdot>)  "<xdot>"
  Igore Initialization Transients (t<=2s)/1(VelFdbk) -> VelFdbk/1
  <DecelZero>/1 -> DecelZero/1
  <DecelHld>/1 -> DecelHld/1
  Unit Conversion/1 -> Signal Specification/1
  Bus Selector/2 -> Unit Conversion/1  "<xdot>"
  Signal Specification/1 -> Compare To Constant3/1

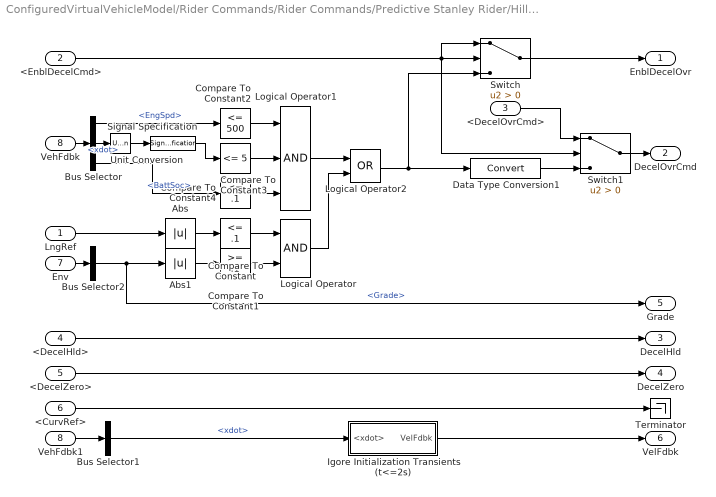
== system ConfiguredVirtualVehicleModel/Rider Commands/Rider Commands/Predictive Stanley Rider/Hill Hold ==
  LngRef : Inport
  <EnblDecelCmd> : Inport  Port=2
  <DecelOvrCmd> : Inport  Port=3
  <DecelHld> : Inport  Port=4
  <DecelZero> : Inport  Port=5
  <CurvRef> : Inport  Port=6
  Env : Inport  Port=7
  VehFdbk : Inport  Port=8
  Abs : Abs  ZeroCross=off  SaturateOnIntegerOverflow=off
  Abs1 : Abs  ZeroCross=off  SaturateOnIntegerOverflow=off
  Bus Selector : BusSelector  OutputSignals=Engine.EngineInfo.EngSpd,Body.BdyFrm.Cg.Vel.xdot,Battery.BattSoc
  Bus Selector1 : BusSelector  OutputSignals=Body.BdyFrm.Cg.Vel.xdot
  Bus Selector2 : BusSelector  OutputSignals=Grade
  Compare To Constant : simulink/Logic and Bit Operations/Compare To Constant  relop=<=  const=.1  OutDataTypeStr=boolean  ZeroCross=off
  Compare To Constant1 : simulink/Logic and Bit Operations/Compare To Constant  relop=>=  const=.1  OutDataTypeStr=boolean  ZeroCross=off
  Compare To Constant2 : simulink/Logic and Bit Operations/Compare To Constant  relop=<=  const=500  OutDataTypeStr=boolean  ZeroCross=off
  Compare To Constant3 : simulink/Logic and Bit Operations/Compare To Constant  relop=<=  const=5  OutDataTypeStr=boolean  ZeroCross=off
  Compare To Constant4 : simulink/Logic and Bit Operations/Compare To Constant  relop=<=  const=.1  OutDataTypeStr=boolean  ZeroCross=off
  Data Type Conversion1 : DataTypeConversion  SaturateOnIntegerOverflow=off  RndMeth=Floor
  Igore Initialization Transients (t<=2s) : Subsystem
  Logical Operator : Logic  AllPortsSameDT=off  OutDataTypeStr=boolean
  Logical Operator1 : Logic  Inputs=3  AllPortsSameDT=off  OutDataTypeStr=boolean
  Logical Operator2 : Logic  Operator=OR  AllPortsSameDT=off  OutDataTypeStr=boolean
  Signal Specification : SignalSpecification  Unit=m/s
  Switch : Switch  Criteria=u2 > Threshold  SaturateOnIntegerOverflow=off  InputSameDT=off
  Switch1 : Switch  Criteria=u2 > Threshold  SaturateOnIntegerOverflow=off  InputSameDT=off
  Terminator : Terminator
  Unit Conversion : UnitConversion
  VehFdbk1 : InportShadow  Port=8
  EnblDecelOvr : Outport
  DecelOvrCmd : Outport  Port=2
  DecelHld : Outport  Port=3
  DecelZero : Outport  Port=4
  Grade : Outport  Port=5
  VelFdbk : Outport  Port=6
  wires:
  Signal Specification/1 -> Compare To Constant3/1
  Bus Selector/2 -> Unit Conversion/1  "<xdot>"
  Unit Conversion/1 -> Signal Specification/1
  <DecelHld>/1 -> DecelHld/1
  <DecelZero>/1 -> DecelZero/1
  VehFdbk1/1 -> Bus Selector1/1
  Bus Selector2/1 -> Abs1/1, Grade/1  "<Grade>"
  Env/1 -> Bus Selector2/1
  Switch1/1 -> DecelOvrCmd/1
  <DecelOvrCmd>/1 -> Switch1/1
  Switch/1 -> EnblDecelOvr/1
  <EnblDecelCmd>/1 -> Switch/2, Switch/1, Switch1/2
  Data Type Conversion1/1 -> Switch1/3
  Bus Selector/3 -> Compare To Constant4/1  "<BattSoc>"
  Bus Selector/1 -> Compare To Constant2/1  "<EngSpd>"
  VehFdbk/1 -> Bus Selector/1
  Compare To Constant4/1 -> Logical Operator1/3
  Logical Operator/1 -> Logical Operator2/2
  Logical Operator1/1 -> Logical Operator2/1
  Compare To Constant3/1 -> Logical Operator1/2
  Compare To Constant2/1 -> Logical Operator1/1
  Compare To Constant1/1 -> Logical Operator/2
  Abs1/1 -> Compare To Constant1/1
  Compare To Constant/1 -> Logical Operator/1
  Abs/1 -> Compare To Constant/1
  Logical Operator2/1 -> Data Type Conversion1/1, Switch/3
  <CurvRef>/1 -> Terminator/1
  LngRef/1 -> Abs/1
  Bus Selector1/1 -> Igore Initialization Transients (t<=2s)/1(<xdot>)  "<xdot>"
  Igore Initialization Transients (t<=2s)/1(VelFdbk) -> VelFdbk/1
